simulink model "MC"  (R2023a)
settings: Solver=FixedStepAuto  StartTime=0.0  StopTime=22.9  RelTol=1e-3
values from neighbouring files (symbols this model uses):
  lujing = 8    [main.m]
libraries: Solver_SF x1
(part 16 of 21)

== matlab function MC/单车道避障参考坐标/纵向滑移量计算模块1 ==
  data: target input; y output
function y  = fcn(target)
y_global=[0	0	0	0	0	0	0	0	0	0	0	0	0	0	0	0	0	0	0	0	0	0	0	0	0	0	0	0	0	0	0	0	0	0	0	0	0	0	0	0	0	0	0	0	0	0	0	0	0	0	0	0	0	0	0	0	0	0	0	0	0	0	0	0	0	0	0	0	0	0	0	0	0	0	0	0	0	0	0	0	0	0	0	0	0	0	0	0	0	0	0	0	0	0	0	0	0	0	0	0	0	0	0	0	0	0	0	0	0	0	0	0	0	0	0	0	0	0	0	0	0	0	0	0	0	0	0	0	0	0	0	0	0	0	0	0	0	0	0	0	0	0	0	0	0	0	0	0	0	0	0	0	0	0	0	0	0	0	0	0	0	0	0	0	0	0	0	0	0	0	0	0	0	0	0	0	0	0	0	0	0	0	0	0	0	0	0	0	0	0	0	0	0	0	0	0	0	0	0	0	0	0	0	0	0	0	0	0	0	0	0	0	0	0	0	0	0	0	0	0	0	0	0	0	0	0	0	0	0	0	0	0	0	0	0	0	0	0	0	0	0	0	0	0	0	0	0	0	0	0	0	0	0	0	0	0	0	0	0	0	0	0	0	0	0	0	0	0	0	0	0	0	0	0	0	0	0	0	0	0	0	0	0	0	0	0	0	0	0	0	0	0	0	0	0	0	0	0	0	0	0	0	0	0	0	0	0	0	0	0	0	0	0	0	0	0	0	0	0	0	0	0	0	0	0	0	0	0	0	0	0	0	0	0	0	0	0	0	0	0	0	0	0	0	0	0	0	0	0	0	0	0	0	0	0	0	0	0	0	0	0	0	0	0	0	0	0	0	0	0	0	0	0	0	0	0	0	0	0	0	0	0	0	0	0	0	0	0	0	0	0	0	0	0	0	0	0	0	0	0	0	0	0	0	0	0	0	0	0	0	0	0	0	0	0	0	0	0	0	0	0	0	0	0	0	0	0	0	0	0	0	0	0	0	0	0	0	0	0	0	0	0	0	0	0	0	0	0	0	0	0	0	0	0	0	0	0	0	0	0	0	0	0	0	0	0	0	0	0	0	0	0	0	0	0	0	0	0	0	0	0	0	0	0	0	0	0	0	0	0	0	0	0	0	0	0	0	0	0	0];
y=0;
if target>length(y_global)-10
    y=1;
end

== matlab function MC/单车道障碍车位置/障碍车1位置 ==
  data: x_obs output; y_obs output; t input
function [x_obs,y_obs] = fcn(t)
N=7;
x_obs=50*ones(N,1);
y_obs=0*ones(N,1);
if t>1
    x_obs=50+10*(t-1)*ones(N,1);
    y_obs=0*ones(N,1);
end

if t>1
    x_obs=50+10*(t-1)*ones(N,1);
    y_obs=0*ones(N,1);
end

== matlab function MC/单车道障碍车位置/障碍车1位置1 ==
  data: x_obs output; y_obs output; t input
function [x_obs,y_obs] = fcn(t)
x_obs=120;
y_obs=1;
if t>1
    x_obs=120+10*(t-1);
    y_obs=1;
end

== matlab function MC/输出路面激励产生的力/模型验证 ==
  data: vy input; output_vx output; output_vy output; output_x output; output_y output; output_theta output; output_phi output; vx input; x input; y input; theta input; phi input; gamma input; dot_phi input; output_gamma output; output_dot_phi output; deltaf input; Fxfl input; Fxfr input; Fxrl input; Fxrr input; thetaf input; thetar input; ax input; zr1 input; zr2 input; zr3 input; zr4 input; zu1 input; zu2 input; zu3 input; zu4 input; d_zs input; zs input; dd_zu1 output; dd_zu2 output; dd_zu3 output; dd_zu4 output; dd_zs output; d_zu1 input; d_zu2 input; d_zu3 input; d_zu4 input; F1 output; F2 output; F3 output; F4 output
function [output_vx,output_vy,output_x,output_y,output_theta,output_phi,output_gamma,output_dot_phi,dd_zu1,dd_zu2,dd_zu3,dd_zu4,dd_zs,F1,F2,F3,F4] = fcn(vy,vx,x,y,theta,phi,gamma,dot_phi,deltaf,Fxfl,Fxfr,Fxrl,Fxrr,thetaf,thetar,ax,zr1,zr2,zr3,zr4,zu1,zu2,zu3,zu4,d_zs,zs,d_zu1,d_zu2,d_zu3,d_zu4)

tf=0.215;
tr=0.215;
d=1.48;
Iz=2059.2;
Ixx=606.6;
% Iy=1536.7;
p=0.5;
Ts=0.001;
lf=1.05;
lr=1.61;
ksfl=27000*0.5;
ksfr=27000*0.5;
ksrl=27000*0.5;
ksrr=27000*0.5;
csfl=1500;
csfr=1500;
csrl=1500;
csrr=1500;

kt1=232000;
kt2=232000;
kt3=232000;
kt4=232000;

m=1430;
ms=1360;
mu1 = 80/2;
mu2= 80/2;
mu3 = 80/2;
mu4= 80/2;
hs=0.315;
h=0.54;
cf=-90700;
cr=-109000;
g=9.8;

kphi=189506*0.1;
cphi=6364;



% thetaf=atan();
% thetar=2;


Mx=tf/2*(-Fxfl+Fxfr)*tan(thetaf)+tr/2*(Fxrl-Fxrr)*tan(thetaf);
My=lf*(Fxfl+Fxfr)*tan(thetaf)+lr*(Fxrr+Fxrl)*tan(thetar);
Mz=tf/2*(-Fxfl+Fxfr)+tr/2*(-Fxrl+Fxrr);
%% 悬架力
zs1=zs+d/2*phi;
zs2=zs-d/2*phi;
zs3=zs+d/2*phi;
zs4=zs-d/2*phi;

d_zs1=d_zs+d/2*dot_phi;
d_zs2=d_zs-d/2*dot_phi;
d_zs3=d_zs+d/2*dot_phi;
d_zs4=d_zs-d/2*dot_phi;

F1=-ksfl*(zs1-zu1)-csfl*(d_zs1-d_zu1);
F2=-ksfr*(zs2-zu2)-csfr*(d_zs2-d_zu2);
F3=-ksrl*(zs3-zu3)-csrl*(d_zs3-d_zu3);
F4=-ksrr*(zs4-zu4)-csrr*(d_zs4-d_zu4);

dd_zs =(F1+F2+F3+F4)/ms;


dd_zu1=(kt1*(zr1-zu1)-F1)/mu1;
dd_zu2=(kt2*(zr2-zu2)-F2)/mu2;
dd_zu3=(kt3*(zr3-zu3)-F3)/mu3;
dd_zu4=(kt4*(zr4-zu4)-F4)/mu4;

% zs=zs;

% F1fl=-ksfl*(zrfl)-csfl*(dot_zrfl);
% F1fr=-ksfr*(zrfr)-csfr*(dot_zrfr);
% F1rl=-ksrl*(zrrl)-csrl*(dot_zrrl);
% F1rr=-ksrr*(zrrr)-csrr*(dot_zrrr);

%% gamma是横摆角速度，psi是俯仰角，phi是侧倾角
alphaf=(vy+lf*gamma)/vx-deltaf;
alphar=(vy-lr*gamma)/vx;
fy=cf*alphaf*2+cr*alphar*2;

dot_vy=-vx*gamma+ms*hs*(kphi-ms*g*hs)/(-ms^2*hs^2+m*Ixx)*phi+ms*hs*cphi/(-ms^2*hs^2+m*Ixx)*dot_phi+Ixx*(fy)/(-ms^2*hs^2+m*Ixx);
dot_gamma=(2*cf*(lf*alphaf)-2*lr*cr*alphar)/Iz;
dot_dot_phi=-m*(kphi-ms*g*hs)/(-ms^2*hs^2+m*Ixx)*phi-m*cphi/(-ms^2*hs^2+m*Ixx)*dot_phi+ms*hs*(fy)/(-ms^2*hs^2+m*Ixx)-(-d/2*(F1+F3)+d/2*(F2+F4))/Ixx;
dot_vx=ax+vy*gamma;
dot_x=vx*cos(theta)-vy*sin(theta);
dot_y=vx*sin(theta)+vy*cos(theta);
% dd_zu1=(kt1*(zr1-zu1)-F1)/mu1;
% dd_zu2=(kt2*(zr2-zu2)-F2)/mu2;
% dd_zu3=(kt3*(zr3-zu3)-F3)/mu3;
% dd_zu4=(kt4*(zr4-zu4)-F4)/mu4;


output_dot_phi=dot_dot_phi*Ts+dot_phi;
output_gamma=dot_gamma*Ts+gamma;
output_phi=dot_phi*Ts+phi;
output_theta=gamma*Ts+theta;
output_vx=dot_vx*Ts+vx;
output_vy=dot_vy*Ts+vy;
output_x=dot_x*Ts+x;
output_y=dot_y*Ts+y;

== matlab function MC/Subsystem/MATLAB Function ==
  data: y input; thetaf output; x input
function thetaf = fcn(y,x)

thetaf = atan(y/x);
end

== matlab function MC/Subsystem/MATLAB Function1 ==
  data: y input; thetaf output; x input
function thetaf = fcn(y,x)

thetaf = atan(y/x);
end
